simulink subsystem "approximate_drag"  (R2024b)
settings: Solver=VariableStepAuto  StartTime=0.0  StopTime=10.0  RelTol=1e-3
undefined symbols (not defined in the file or in its folder): DRAG_DATA, PLATE_AREA, PLATE_CD, REF_AREA
settings Model: Creator=yevge  LastModifiedBy=yevge

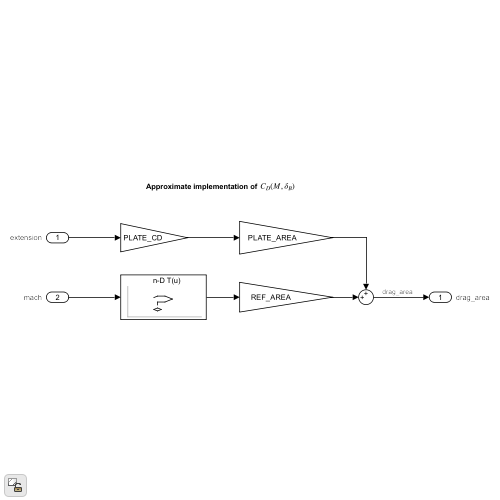
[thumbnail: Simulink's stored preview of the top-level diagram]
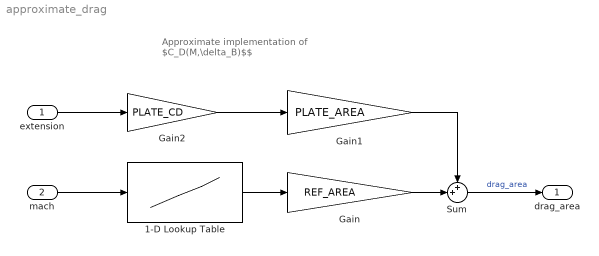
== system approximate_drag ==
  note: Approximate implementation of $C_D(M,\delta_B)$$
  extension : Inport  OutMin=0  OutMax=1  Unit=1  PortDimensions=1
  mach : Inport  Port=2  Unit=1  PortDimensions=1
  1-D Lookup Table : Lookup_n-D  NumberOfTableDimensions=1  BreakpointsForDimension1=DRAG_DATA.MACH  Table=DRAG_DATA.DRAG  ExtrapMethod=Clip  UseLastTableValue=on  InternalRulePriority=Speed  RndMeth=Simplest
  Gain : Gain  Gain=REF_AREA
  Gain1 : Gain  Gain=PLATE_AREA
  Gain2 : Gain  Gain=PLATE_CD
  Sum : Sum  Inputs=++|
  drag_area : Outport  Unit=m^2  PortDimensions=1
  wires:
  Gain1/1 -> Sum/1
  Gain2/1 -> Gain1/1
  1-D Lookup Table/1 -> Gain/1
  Sum/1 -> drag_area/1  "drag_area"
  Gain/1 -> Sum/2
  mach/1 -> 1-D Lookup Table/1
  extension/1 -> Gain2/1
